simulink model "MPTC_conventional"  (R2019b)
settings: Solver=ode4  StartTime=0.0  StopTime=1  FixedStep=50e-6  RelTol=1e-3  EnableMultiTasking=on
values from neighbouring files (symbols this model uses):
  B = 0    [Parameters_MPC.m]
  J = 0.0165    [Parameters_MPC.m]
  kr = (Lm/Lr)    (= 0.960714285714)    [Parameters_MPC.m]
  Lm = 0.0538    [Parameters_MPC.m]
  P = 2    [Parameters_MPC.m]
  r_sigma = Rs+Rr*(kr^2)    (= 0.445903864796)    [Parameters_MPC.m]
  Rs = 0.277    [Parameters_MPC.m]
  set_speed = 500    [Parameters_MPC.m]
  t_sigma = (sigma*Ls)/(r_sigma)    (= 0.00810392489023)    [Parameters_MPC.m]
  tr = Lr/Rr    (= 0.306010928962)    [Parameters_MPC.m]
libraries: powerlib_meascontrol x4, simulink x2, powerlib x1
settings Model: Creator=91913  LastModifiedBy=akhil
settings SolverCC: PositivePriorityOrder=on  AutoInsertRateTranBlk=on
settings DataIOCC: SaveFormat=StructureWithTime  SaveOutput=off  DSMLogging=off  ReturnWorkspaceOutputs=off  SignalLoggingName=logsout_MPTC

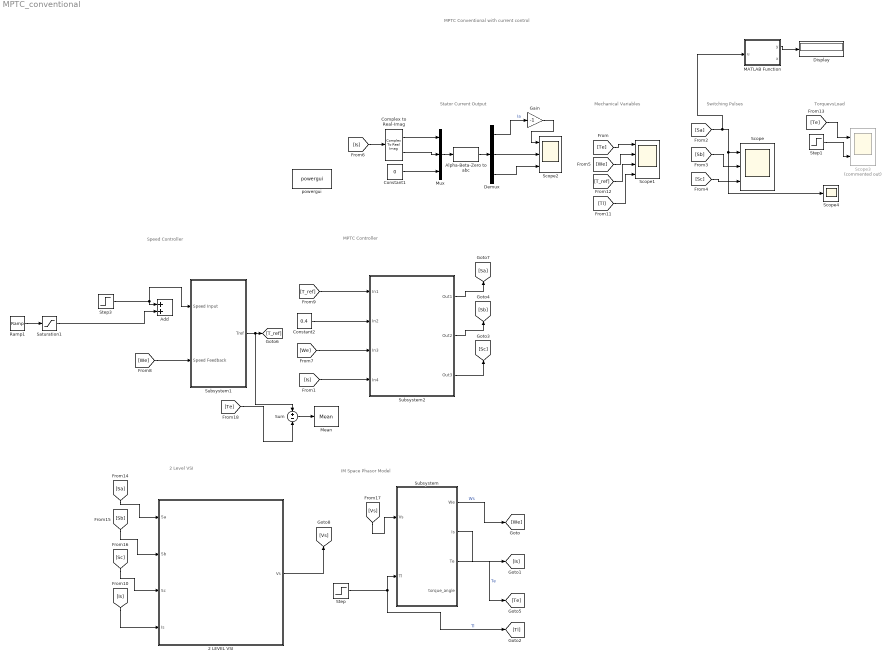
== system MPTC_conventional ==
  note: MPTC Conventional with current control
  note: Mechanical Variables
  note: Switching Pulses
  note: Speed Controller
  note: 2 Level VSI
  note: MPTC Controller
  note: IM Space Phasor Model
  note: Stator Current Output
  note: TorquevsLoad
  2 LEVEL VSI : Subsystem
  Add : Sum
  Alpha-Beta-Zero to abc : powerlib_meascontrol/Transformations/Alpha-Beta-Zero to abc
      settings: SourceProductName=Simscape Electrical  SourceProductBaseCode=PS
  Complex to Real-Imag : ComplexToRealImag
  Constant1 : Constant  Value=0
  Constant2 : Constant  Value=0.4
  Demux : Demux  Outputs=3
  Display : Display
  Gain : Gain  Gain=-1
  MATLAB Function : MATLAB Function  TreatAsAtomicUnit=on
  Mean : powerlib_meascontrol/Measurements/Mean  Freq=40  Vinit=0  Ts=0
      settings: SourceProductName=Simscape Electrical
  Mux : Mux  Inputs=3
  Ramp1 : simulink/Sources/Ramp  slope=-2*set_speed  start=0.4  InitialOutput=0
  Saturation1 : Saturate  UpperLimit=0  LowerLimit=-200
  Scope : Scope  NumInputPorts=3
  Scope1 : Scope  NumInputPorts=4
  Scope2 : Scope  NumInputPorts=3
  Scope3 : Scope  Commented=on  NumInputPorts=2
  Scope4 : Scope
  Step : Step  Time=0.5  After=20  SampleTime=0
  Step1 : Step  Time=1.5  After=20  SampleTime=0
  Step3 : Step  Time=0.1  After=set_speed  SampleTime=0
  Subsystem : Subsystem
  Subsystem1 : Subsystem
      mask Display: image('C:\Users\91913\OneDrive\Desktop\Comparisons\Speed_Track_MPTCTR.jpg'); % Use "Edit Image" on toolstrip to change.
  Subsystem2 : Subsystem
      mask Display: image('C:\Users\91913\OneDrive\Desktop\Presentation_Figures\MPTC_Scheme.JPG'); % Use "Edit Image" on toolstrip to change.
  Sum : Sum  Inputs=+-
  powergui : powerlib/powergui  Priority=1  SimulationMode=Continuous  SampleTime=50e-6  frequency=60  Iterations=50  frequencyindice=60  Pbase=100e6  ErrMax=1e-4  UnitsV=kV  UnitsW=MW  buscounter=0  FunctionMessages=off  echomessages=off  EnableUseOfTLC=off  CurrentSourceSwitches=off  DisableSnubberDevices=off  DisableRonSwitches=off  DisableVfSwitches=off  DisplayEquations=off  AutomaticDiscreteSolvers=off  SolverType=Tustin/Backward Euler (TBE)  Interpol=off  ExternalGateDelay=off  methode=off  Ts=100  x0status=blocks  SPID=on  SwTol=0  HookPort=off  NonlinearTolerance=1e-4  nMaxIteration=100  ContinueOnMaxIteration=off  RestoreLinks=warning  ResistiveCurrentMeasurement=off  Frange=[0:2:500]  Ylog=off  Xlog=on  ShowGrid=off  save=off  variable=ZData  structure=logsout  ZoomFFT=off  StartTime=3  cycles=50  DisplayStyle=1  fundamental=10.86  FreqAxis=off  MaxFrequency=1000  frequencyindicesteady=1  RmsSteady=1  display=off
      settings: SourceProductName=Simscape Electrical
  wires:
  Subsystem/1(We) -> [We]  "Ws"
  Subsystem/2(Is) -> [Is]
  [Sa] -> MATLAB Function/1(u), Scope4/1, Scope/1
  [Sb] -> Scope/2
  [Sc] -> Scope/3
  Subsystem/3(Te) -> [Te]  "Te"
  [Te] -> Scope1/1
  [We] -> Scope1/2
  [Is] -> Complex to Real-Imag/1
  Complex to Real-Imag/2 -> Mux/2
  Constant1/1 -> Mux/3
  Mux/1 -> Alpha-Beta-Zero to abc/1
  Complex to Real-Imag/1 -> Mux/1
  Alpha-Beta-Zero to abc/1 -> Demux/1
  Demux/2 -> Scope2/2
  [We] -> Subsystem1/2(Speed Feedback)
  Subsystem1/1(Tref) -> Sum/1, [T_ref]
  [T_ref] -> Scope1/3
  Constant2/1 -> Subsystem2/2(In2)
  [We] -> Subsystem2/3(In3)
  [Is] -> Subsystem2/4(In4)
  Demux/3 -> Scope2/3
  [Is] -> 2 LEVEL VSI/4(Is)
  [Tl] -> Scope1/4
  [Te] -> Scope3/1
  Step1/1 -> Scope3/2
  Subsystem2/1(Out1) -> [Sa]
  Subsystem2/3(Out3) -> [Sc]
  Subsystem2/2(Out2) -> [Sb]
  [Sc] -> 2 LEVEL VSI/3(Sc)
  [Sa] -> 2 LEVEL VSI/1(Sa)
  [Sb] -> 2 LEVEL VSI/2(Sb)
  2 LEVEL VSI/1(Vs) -> [Vs]
  [Vs] -> Subsystem/1(Vs)
  [Te] -> Sum/2
  Sum/1 -> Mean/1
  [T_ref] -> Subsystem2/1(In1)
  Demux/1 -> Gain/1  "Ia"
  Gain/1 -> Scope2/1
  Step/1 -> [Tl], Subsystem/2(Tl)  "Tl"
  MATLAB Function/1(y) -> Display/1
  Ramp1/1 -> Saturation1/1
  Step3/1 -> Add/1, Subsystem1/1(Speed Input)
  Saturation1/1 -> Add/2

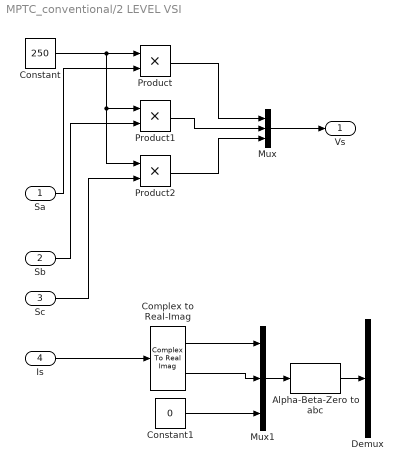
== system MPTC_conventional/2 LEVEL VSI ==
  Sa : Inport
  Sb : Inport  Port=2
  Sc : Inport  Port=3
  Is : Inport  Port=4
  Alpha-Beta-Zero to abc : powerlib_meascontrol/Transformations/Alpha-Beta-Zero to abc
      settings: SourceProductName=Simscape Electrical  SourceProductBaseCode=PS
  Complex to Real-Imag : ComplexToRealImag
  Constant : Constant  Value=250
  Constant1 : Constant  Value=0
  Demux : Demux  Outputs=3
  Mux : Mux  Inputs=3
  Mux1 : Mux  Inputs=3
  Product : Product
  Product1 : Product
  Product2 : Product
  Vs : Outport
  wires:
  Sa/1 -> Product/2
  Sb/1 -> Product1/2
  Sc/1 -> Product2/2
  Constant/1 -> Product2/1, Product1/1, Product/1
  Product/1 -> Mux/1
  Product1/1 -> Mux/2
  Product2/1 -> Mux/3
  Mux/1 -> Vs/1
  Alpha-Beta-Zero to abc/1 -> Demux/1
  Complex to Real-Imag/1 -> Mux1/1
  Complex to Real-Imag/2 -> Mux1/2
  Constant1/1 -> Mux1/3
  Mux1/1 -> Alpha-Beta-Zero to abc/1
  Is/1 -> Complex to Real-Imag/1

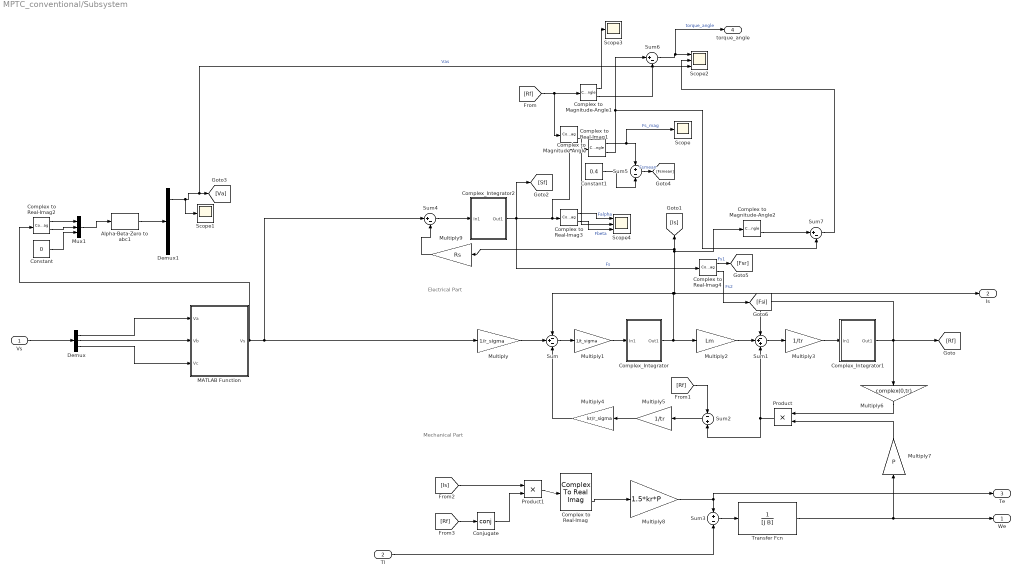
== system MPTC_conventional/Subsystem ==
  note: Mechanical Part
  note: Electrical Part
  Vs : Inport
  Tl : Inport  Port=2
  Alpha-Beta-Zero to abc1 : powerlib_meascontrol/Transformations/Alpha-Beta-Zero to abc
      settings: SourceProductName=Simscape Electrical  SourceProductBaseCode=PS
  Complex to Magnitude-Angle : ComplexToMagnitudeAngle
  Complex to Magnitude-Angle1 : ComplexToMagnitudeAngle
  Complex to Magnitude-Angle2 : ComplexToMagnitudeAngle
  Complex to Real-Imag{,1..4} (5 alike) : ComplexToRealImag
  Complex_Integrator : Subsystem
  Complex_Integrator1 : Subsystem
  Complex_Integrator2 : Subsystem
  Conjugate : Math  Operator=conj  RndMeth=Zero  SaturateOnIntegerOverflow=on
  Constant : Constant  Value=0
  Constant1 : Constant  Value=0.4
  Demux : Demux  Outputs=3
  Demux1 : Demux  Outputs=3
  MATLAB Function : MATLAB Function  TreatAsAtomicUnit=on
  Multiply : Gain  Gain=1/r_sigma
  Multiply1 : Gain  Gain=1/t_sigma
  Multiply2 : Gain  Gain=Lm
  Multiply3 : Gain  Gain=1/tr
  Multiply4 : Gain  Gain=kr/r_sigma
  Multiply5 : Gain  Gain=1/tr
  Multiply6 : Gain  Gain=complex(0,tr)
  Multiply7 : Gain  Gain=P
  Multiply8 : Gain  Gain=1.5*kr*P
  Multiply9 : Gain  Gain=Rs
  Mux1 : Mux  Inputs=3
  Product : Product
  Product1 : Product
  Scope : Scope
  Scope1 : Scope
  Scope2 : Scope  NumInputPorts=3
  Scope3 : Scope
  Scope4 : Scope  NumInputPorts=3
  Sum : Sum  Inputs=-+-
  Sum1 : Sum  Inputs=-++
  Sum2 : Sum  Inputs=-+
  Sum3 : Sum  Inputs=+-
  Sum4 : Sum  Inputs=|+-
  Sum5 : Sum  Inputs=+-
  Sum6 : Sum  Inputs=|+-
  Sum7 : Sum  Inputs=|+-
  Transfer Fcn : TransferFcn  Denominator=[J B]
  We : Outport
  Is : Outport  Port=2
  Te : Outport  Port=3
  torque_angle : Outport  Port=4
  wires:
  [Is] -> Product1/1
  Multiply1/1 -> Complex_Integrator/1(In1)
  Multiply4/1 -> Sum/3
  Multiply3/1 -> Complex_Integrator1/1(In1)
  Sum1/1 -> Multiply3/1
  Complex to Real-Imag/2 -> Multiply8/1
  Complex_Integrator1/1(Out1) -> Sum1/1, [Rf], Multiply6/1
  Tl/1 -> Sum3/2
  Conjugate/1 -> Product1/2
  Multiply7/1 -> Product/2
  Multiply8/1 -> Sum3/1, Te/1
  Multiply2/1 -> Sum1/2
  Multiply/1 -> Sum/2
  Multiply6/1 -> Product/1
  Product/1 -> Sum2/2, Sum1/3
  Multiply5/1 -> Multiply4/1
  Sum2/1 -> Multiply5/1
  Transfer Fcn/1 -> We/1, Multiply7/1
  Sum/1 -> Multiply1/1
  [Rf] -> Conjugate/1
  Product1/1 -> Complex to Real-Imag/1
  Sum3/1 -> Transfer Fcn/1
  [Rf] -> Sum2/1
  Sum4/1 -> Complex_Integrator2/1(In1)
  Complex_Integrator2/1(Out1) -> Complex to Real-Imag4/1, Complex to Magnitude-Angle/1, Complex to Real-Imag3/1, [Sf]  "Fs"
  Multiply9/1 -> Sum4/2
  Complex_Integrator/1(Out1) -> Multiply2/1, Complex to Magnitude-Angle2/1, Multiply9/1, [Is], Is/1, Sum/1
  MATLAB Function/1(Vs) -> Complex to Real-Imag2/1, Sum4/1, Multiply/1
  Vs/1 -> Demux/1
  Demux/1 -> MATLAB Function/1(Va)
  Demux/2 -> MATLAB Function/2(Vb)
  Demux/3 -> MATLAB Function/3(Vc)
  Constant/1 -> Mux1/3
  Alpha-Beta-Zero to abc1/1 -> Demux1/1
  Mux1/1 -> Alpha-Beta-Zero to abc1/1
  Complex to Real-Imag2/2 -> Mux1/2
  Complex to Real-Imag2/1 -> Mux1/1
  Demux1/1 -> Scope1/1, Scope2/3, [Va]  "Vas"
  Complex to Magnitude-Angle/1 -> Scope/1, Sum5/1  "Fs_mag"
  Constant1/1 -> Sum5/2
  Sum5/1 -> [Fsmean]  "Fsmean"
  [Rf] -> Complex to Real-Imag1/1, Complex to Magnitude-Angle1/1
  Complex to Magnitude-Angle1/2 -> Sum6/2
  Complex to Magnitude-Angle/2 -> Sum7/2, Sum6/1
  Sum6/1 -> torque_angle/1, Scope2/1  "torque_angle"
  Complex to Magnitude-Angle1/1 -> Scope3/1
  Complex to Magnitude-Angle2/2 -> Sum7/1
  Sum7/1 -> Scope2/2
  Complex to Real-Imag3/2 -> Scope4/3  "Fbeta"
  Complex to Real-Imag1/2 -> Scope4/2
  Complex to Real-Imag3/1 -> Scope4/1  "Falpha"
  Complex to Real-Imag4/2 -> [Fsi]  "Fs2"
  Complex to Real-Imag4/1 -> [Fsr]  "Fs1"

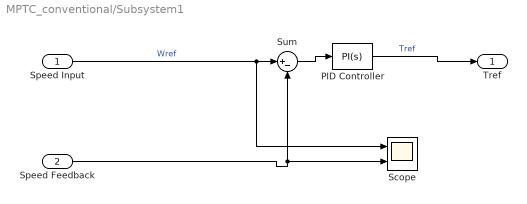
== system MPTC_conventional/Subsystem1 ==
  Speed Input : Inport
  Speed Feedback : Inport  Port=2
  PID Controller : simulink/Continuous/PID Controller  Controller=PI  Form=Parallel  TimeDomain=Continuous-time  SampleTime=-1  IntegratorMethod=Forward Euler  FilterMethod=Forward Euler  ControllerParametersSource=internal  P=100  I=2000  D=0  UseFilter=on  N=100  TunerSelectOption=Transfer Function Based (PID Tuner App)  InitialConditionSource=internal  InitialConditionForIntegrator=0  InitialConditionForFilter=0  DifferentiatorICPrevScaledInput=0  ExternalReset=none  TrackingMode=off  Kt=1  LimitOutput=on  UpperSaturationLimit=30  LowerSaturationLimit=-30  LinearizeAsGain=on  AntiWindupMode=clamping  Kb=0.9  POutMin=[]  POutMax=[]  IOutMin=[]  IOutMax=[]  DOutMin=[]  DOutMax=[]  NOutMin=[]  NOutMax=[]  SumOutMin=[]  SumOutMax=[]  SaturationOutMin=[]  SaturationOutMax=[]  PParamMin=[]  PParamMax=[]  IParamMin=[]  IParamMax=[]  DParamMin=[]  DParamMax=[]  NParamMin=[]  NParamMax=[]  KbParamMin=[]  KbParamMax=[]  KtParamMin=[]  KtParamMax=[]  KbOutMin=[]  KbOutMax=[]  KtOutMin=[]  KtOutMax=[]  IntegratorOutMin=[]  IntegratorOutMax=[]  FilterOutMin=[]  FilterOutMax=[]  SumI1OutMin=[]  SumI1OutMax=[]  SumI2OutMin=[]  SumI2OutMax=[]  SumI3OutMin=[]  SumI3OutMax=[]  SumI4OutMin=[]  SumI4OutMax=[]  SumDOutMin=[]  SumDOutMax=[]  DifferentiatorOutMin=[]  DifferentiatorOutMax=[]  FilterDiffOutCoefMin=[]  FilterDiffOutCoefMax=[]  ReciprocalOutMin=[]  ReciprocalOutMax=[]  SumDenOutMin=[]  SumDenOutMax=[]  SumNumOutMin=[]  SumNumOutMax=[]  DivideOutMin=[]  DivideOutMax=[]  IntegratorContinuousStateAttributes=''  IntegratorStateMustResolveToSignalObject=off  IntegratorRTWStateStorageClass=Auto  FilterContinuousStateAttributes=''  FilterStateMustResolveToSignalObject=off  FilterRTWStateStorageClass=Auto  ParallelPVariant=InternalParameters  IdealPVariant=Disabled  IVariant=InternalParameters  DVariant=Disabled  IntegratorVariant=Continuous  SatVariant=Enabled  AWVariant=ContClampingParallel  PCopyVariant=Disabled  TRVariant=Disabled  FdbkBlocksVariant=Forward  IdealPFdbkVariant=Disabled  SatFdbkVariant=Disabled  DerivativeFilterVariant=Disabled  NVariant=Disabled  NCopyVariant=Disabled_SignalSpec  FilterICVariant=Disabled  IntegratorICVariant=InternalICs  ExternalResetVariant=Disabled  TRSumVariant=Passthrough  SumFdbkVariant=Disabled  SumVariant=Sum_PI
  Scope : Scope  NumInputPorts=2
  Sum : Sum  Inputs=|+-
  Tref : Outport
  wires:
  Speed Input/1 -> Scope/1, Sum/1  "Wref"
  Speed Feedback/1 -> Sum/2, Scope/2
  Sum/1 -> PID Controller/1
  PID Controller/1 -> Tref/1  "Tref"

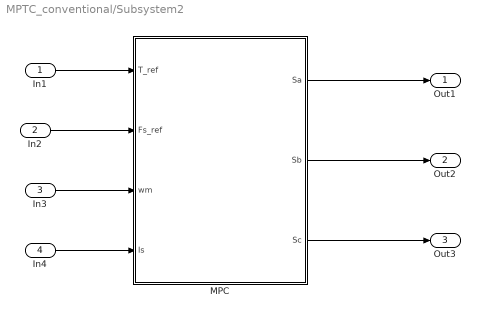
== system MPTC_conventional/Subsystem2 ==
  In1 : Inport
  In2 : Inport  Port=2
  In3 : Inport  Port=3
  In4 : Inport  Port=4
  MPC : MATLAB Function  TreatAsAtomicUnit=on
  Out1 : Outport
  Out2 : Outport  Port=2
  Out3 : Outport  Port=3
  wires:
  In4/1 -> MPC/4(Is)
  In3/1 -> MPC/3(wm)
  MPC/2(Sb) -> Out2/1
  MPC/1(Sa) -> Out1/1
  MPC/3(Sc) -> Out3/1
  In1/1 -> MPC/1(T_ref)
  In2/1 -> MPC/2(Fs_ref)

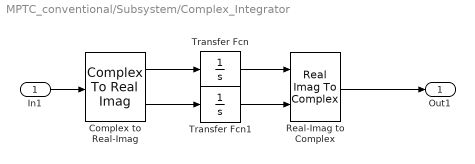
== system MPTC_conventional/Subsystem/Complex_Integrator ==
  In1 : Inport
  Complex to Real-Imag : ComplexToRealImag
  Real-Imag to Complex : RealImagToComplex
  Transfer Fcn : TransferFcn  Denominator=[1 0]
  Transfer Fcn1 : TransferFcn  Denominator=[1 0]
  Out1 : Outport
  wires:
  In1/1 -> Complex to Real-Imag/1
  Complex to Real-Imag/1 -> Transfer Fcn/1
  Complex to Real-Imag/2 -> Transfer Fcn1/1
  Transfer Fcn/1 -> Real-Imag to Complex/1
  Transfer Fcn1/1 -> Real-Imag to Complex/2
  Real-Imag to Complex/1 -> Out1/1

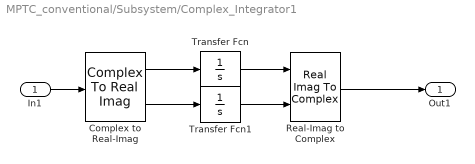
== system MPTC_conventional/Subsystem/Complex_Integrator1 ==
  In1 : Inport
  Complex to Real-Imag : ComplexToRealImag
  Real-Imag to Complex : RealImagToComplex
  Transfer Fcn : TransferFcn  Denominator=[1 0]
  Transfer Fcn1 : TransferFcn  Denominator=[1 0]
  Out1 : Outport
  wires:
  In1/1 -> Complex to Real-Imag/1
  Complex to Real-Imag/1 -> Transfer Fcn/1
  Complex to Real-Imag/2 -> Transfer Fcn1/1
  Transfer Fcn/1 -> Real-Imag to Complex/1
  Transfer Fcn1/1 -> Real-Imag to Complex/2
  Real-Imag to Complex/1 -> Out1/1

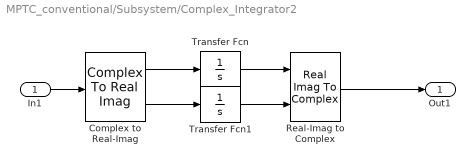
== system MPTC_conventional/Subsystem/Complex_Integrator2 ==
  In1 : Inport
  Complex to Real-Imag : ComplexToRealImag
  Real-Imag to Complex : RealImagToComplex
  Transfer Fcn : TransferFcn  Denominator=[1 0]
  Transfer Fcn1 : TransferFcn  Denominator=[1 0]
  Out1 : Outport
  wires:
  In1/1 -> Complex to Real-Imag/1
  Complex to Real-Imag/1 -> Transfer Fcn/1
  Complex to Real-Imag/2 -> Transfer Fcn1/1
  Transfer Fcn/1 -> Real-Imag to Complex/1
  Transfer Fcn1/1 -> Real-Imag to Complex/2
  Real-Imag to Complex/1 -> Out1/1

== matlab function MPTC_conventional/Subsystem2/MPC ==
  settings: updateMethod=DISCRETE
  data: T_ref input; Sa output; Fs_ref input; wm input; Is input; Sb output; Sc output
function [Sa,Sb,Sc]   = MPC(T_ref,Fs_ref,wm,Is)

Ts=50e-6;%Sampling time or Time Window for Kth sample
%Supply DC Voltage
Vdc=250;
%Machine Parameters
Rs=0.277;
Rr=0.183;
Lr=0.056;
Ls=0.0553;
Lm=0.0538;
P=2;%pole pairs
T_nom=25;
Is_nom=25;
%Electrical Time Constants
tr=Lr/Rr;
%Constants in equation
sigma=(1-(Lm^2)/(Ls*Lr));
kr=(Lm/Lr);
r_sigma=Rs+Rr*(kr^2);
t_sigma=(sigma*Ls)/(r_sigma);


%Voltage vectors
V0=0;
V1=complex((2/3)*Vdc,0);
V2=complex((1/3)*Vdc,(sqrt(3)/3)*Vdc);
V3=complex((-1/3)*Vdc,(sqrt(3)/3)*Vdc);
V4=-V1;
V5=-V2;
V6=-V3;
V7= V0;
V=[V0 V1 V2 V3 V4 V5 V6 V7];
%Switching States
cost_opt=1e14;
states=[0 0 0;1 0 0;1 1 0;0 1 0;0 1 1;0 0 1;1 0 1;1 1 1];

persistent x_opt Fs%since previous values are required for prediction and estimation
if isempty(x_opt)
    x_opt=1;
end
if isempty(Fs)
    Fs=complex(0,0);
end

%stator flux estimate
Fs=Fs+Ts*(V(x_opt)-(Rs*Is));
%Rotor Flux estimate
Fr=(Lr/Lm)*Fs+Is*(Lm-(Lr*Ls/Lm));

%Prediction of stator current,flux vectors and Torque for each voltage
%vectors

for loop=1:8
    
    V_loop=V(loop);% iterative voltage vector
    %Stator flux prediction based on discretization
    Fsp=Fs+(Ts*V_loop)-Rs*Ts*Is;
    %Stator current prediction
    Isp=Is*(t_sigma/(Ts+t_sigma))+(Ts/(t_sigma+Ts))*(1/r_sigma)*(Fr*((kr/tr)-complex(0,wm*kr))+V_loop);
    %Torque prediction
    Tp=(3/2)*P*imag(conj(Fsp)*Isp);
    %Cost Function
     cost=1.25*(abs(T_ref-Tp)/T_nom)+5*(abs(Fs_ref-abs(Fsp))/Fs_ref);

     if(cost<cost_opt) 
     x_opt=loop;
     cost_opt=cost;
     end    
     if ( abs(real(Is)) > Is_nom )
           x_opt=1;
     end
     
end
%Outpt switching states
Sa=states(x_opt,1);
Sb=states(x_opt,2);
Sc=states(x_opt,3);

== matlab function MPTC_conventional/Subsystem/MATLAB Function ==
  data: Va input; Vs output; Vb input; Vc input
function Vs = fcn(Va,Vb,Vc)

a=complex(cos(2*pi/3),sin(2*pi/3)); 
Vs =(2/3)*(Va+(a*Vb)+((a^2)*Vc)) ;

== matlab function MPTC_conventional/MATLAB Function ==
  settings: updateMethod=DISCRETE
  data: u input; y output; x output
function [y,x] = fcn(u)
x=5;
persistent count prestate;
if(isempty(count))
    count=0;
end    
if(isempty(prestate))
    prestate=0;
end  
if(u~=prestate)
count=count+1; 
x=100;
else
x=-100;    
end

prestate=u;


y=count;
